simulink model "overcurrent_undervoltag_relay"  (R2025b)
settings: Solver=VariableStepAuto  StartTime=0.0  StopTime=2.00  RelTol=1e-3
libraries: dspstat3 x3, simulink x1
settings Model: Creator=urshi  LastModifiedBy=urshi

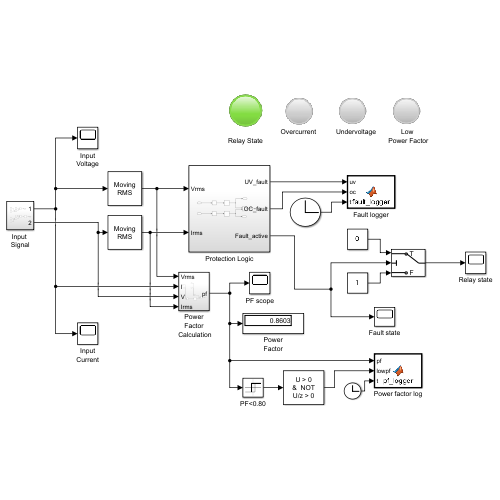
[thumbnail: Simulink's stored preview of the top-level diagram]
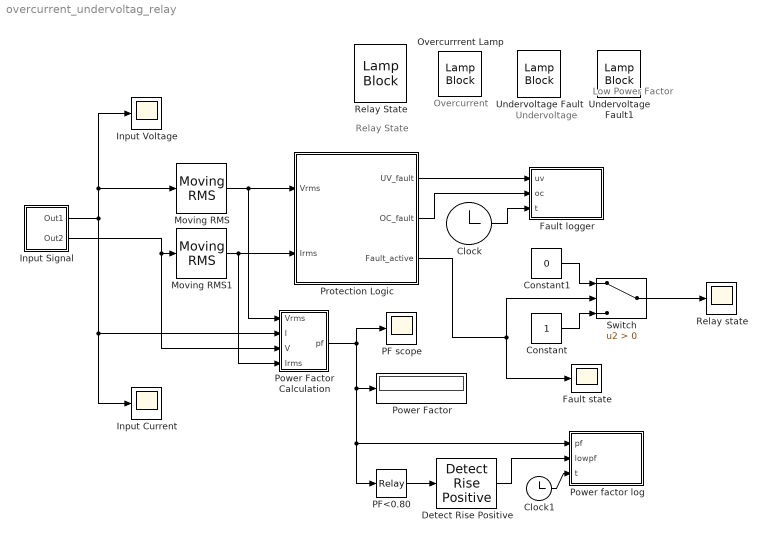
== system overcurrent_undervoltag_relay ==
  note: Low
      | Power Factor
  note: Relay State
  note: Undervoltage
  note: Overcurrent
  Clock : Clock
  Clock1 : Clock
  Constant : Constant
  Constant1 : Constant  Value=0
  Detect Rise Positive : simulink/Logic and Bit Operations/Detect Rise Positive  vinit=0  OutDataTypeStr=boolean
  Fault logger : MATLAB Function  TreatAsAtomicUnit=on
  Fault state : Scope
      settings: ActiveDisplayYMinimum=-6.1678141135617093  ActiveDisplayYMaximum=11.611256622792828  DataLoggingVariableName=ScopeData2
  Input Current : Scope
      settings: ActiveDisplayYMinimum=-1422.9675846946514  ActiveDisplayYMaximum=1324.8355096908929
  Input Voltage : Scope
      settings: ActiveDisplayYMinimum=-1422.9675846946514  ActiveDisplayYMaximum=1324.8355096908929
  Input Signal : Subsystem
  Moving RMS : dspstat3/Moving RMS  Method=Sliding window  ForgettingFactorPort=off  SpecifyWindowLength=on  WindowLength=200  OverlapLength=199  AllowArbitraryInputLength=off  ForgettingFactor=0.9  SimulateUsing=Interpreted execution
  Moving RMS1 : dspstat3/Moving RMS  Method=Sliding window  ForgettingFactorPort=off  SpecifyWindowLength=on  WindowLength=200  OverlapLength=199  AllowArbitraryInputLength=off  ForgettingFactor=0.9  SimulateUsing=Interpreted execution
  Overcurrrent Lamp : LampBlock  LabelPosition=Hide  DefaultColor=[192.0, 192.0, 192.0]
  PF scope : Scope
      settings: ActiveDisplayYMinimum=0.59741062696120162  ActiveDisplayYMaximum=1.1022229106822319  DataLoggingVariableName=ScopeData4
  PF<0.80 : Relay  OnSwitchValue=0.85  OffSwitchValue=0.80  OnOutputValue=0  OffOutputValue=1
  Power Factor : Display
  Power Factor Calculation : Subsystem
  Power factor log : MATLAB Function  TreatAsAtomicUnit=on
  Protection Logic : Subsystem
  Relay State : LampBlock  LabelPosition=Hide  DefaultColor=[192.0, 192.0, 192.0]
  Relay state : Scope
      settings: ActiveDisplayYMinimum=-0.2045815584191954  ActiveDisplayYMaximum=1.4705379923620556  DataLoggingVariableName=ScopeData3
  Switch : Switch  Criteria=u2 > Threshold  SaturateOnIntegerOverflow=off  InputSameDT=off
  Undervoltage Fault : LampBlock  LabelPosition=Hide  DefaultColor=[192.0, 192.0, 192.0]
  Undervoltage Fault1 : LampBlock  LabelPosition=Hide  DefaultColor=[192.0, 192.0, 192.0]
  wires:
  Input Signal/1(Out1) -> Input Voltage/1, Moving RMS/1, Input Current/1, Power Factor Calculation/2(I)
  Moving RMS/1 -> Power Factor Calculation/1(Vrms), Protection Logic/1(Vrms)
  Moving RMS1/1 -> Power Factor Calculation/4(Irms), Protection Logic/2(Irms)
  Protection Logic/1(UV_fault) -> Fault logger/1(uv)
  Protection Logic/2(OC_fault) -> Fault logger/2(oc)
  Clock/1 -> Fault logger/3(t)
  Protection Logic/3(Fault_active) -> Switch/2, Fault state/1
  Constant1/1 -> Switch/1
  Constant/1 -> Switch/3
  Switch/1 -> Relay state/1
  Clock1/1 -> Power factor log/3(t)
  Power Factor Calculation/1(pf) -> Power factor log/1(pf), PF<0.80/1, Power Factor/1, PF scope/1
  Input Signal/2(Out2) -> Power Factor Calculation/3(V), Moving RMS1/1
  Detect Rise Positive/1 -> Power factor log/2(lowpf)
  PF<0.80/1 -> Detect Rise Positive/1

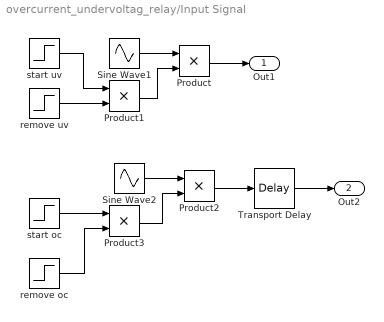
== system overcurrent_undervoltag_relay/Input Signal ==
  Product{,1..3} (4 alike) : Product
  Sine Wave1 : Sin  Amplitude=325.269  Frequency=50*2*pi  SampleTime=0.0002
  Sine Wave2 : Sin  Amplitude=7.071  Frequency=50*2*pi  SampleTime=0.0002
  Transport Delay : TransportDelay  DelayTime=0.00167
  remove oc : Step  Time=0.40  Before=1  After=0.25  SampleTime=0.0002
  remove uv : Step  Time=1.2  Before=1  After=2  SampleTime=0.0002
  start oc : Step  Time=0.15  Before=1  After=4  SampleTime=0.0002
  start uv : Step  Time=0.80  Before=1  After=0.5  SampleTime=0.0002
  Out1 : Outport
  Out2 : Outport  Port=2
  wires:
  remove oc/1 -> Product3/2
  start uv/1 -> Product1/1
  Product3/1 -> Product2/2
  remove uv/1 -> Product1/2
  start oc/1 -> Product3/1
  Product/1 -> Out1/1
  Sine Wave2/1 -> Product2/1
  Sine Wave1/1 -> Product/1
  Product1/1 -> Product/2
  Product2/1 -> Transport Delay/1
  Transport Delay/1 -> Out2/1

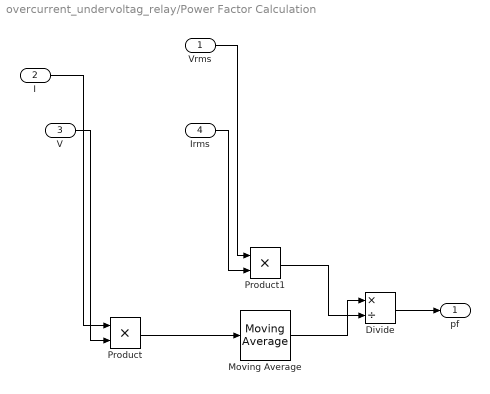
== system overcurrent_undervoltag_relay/Power Factor Calculation ==
  Vrms : Inport
  I : Inport  Port=2
  V : Inport  Port=3
  Irms : Inport  Port=4
  Divide : Product  Inputs=*/
  Moving Average : dspstat3/Moving Average  Method=Sliding window  ForgettingFactorPort=off  SpecifyWindowLength=on  WindowLength=200  OverlapLength=199  AllowArbitraryInputLength=off  ForgettingFactor=0.9  SimulateUsing=Interpreted execution
  Product : Product
  Product1 : Product
  pf : Outport
  wires:
  I/1 -> Product/1
  V/1 -> Product/2
  Divide/1 -> pf/1
  Product/1 -> Moving Average/1
  Moving Average/1 -> Divide/1
  Vrms/1 -> Product1/1
  Irms/1 -> Product1/2
  Product1/1 -> Divide/2

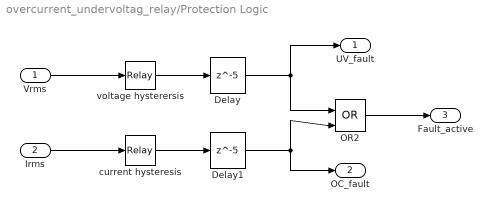
== system overcurrent_undervoltag_relay/Protection Logic ==
  Vrms : Inport
  Irms : Inport  Port=2
  Delay : Delay  DelayLength=5  InputProcessing=Columns as channels (frame based)
  Delay1 : Delay  DelayLength=5  InputProcessing=Columns as channels (frame based)
  OR2 : Logic  Operator=OR  IconShape=distinctive  AllPortsSameDT=off  OutDataTypeStr=boolean
  current hysteresis : Relay  OnSwitchValue=8  OffSwitchValue=7.2
  voltage hysterersis : Relay  OnSwitchValue=190  OffSwitchValue=180  OnOutputValue=0  OffOutputValue=1
  UV_fault : Outport
  OC_fault : Outport  Port=2
  Fault_active : Outport  Port=3
  wires:
  Irms/1 -> current hysteresis/1
  Vrms/1 -> voltage hysterersis/1
  current hysteresis/1 -> Delay1/1
  OR2/1 -> Fault_active/1
  voltage hysterersis/1 -> Delay/1
  Delay/1 -> UV_fault/1, OR2/1
  Delay1/1 -> OR2/2, OC_fault/1

== matlab function overcurrent_undervoltag_relay/Power factor log ==
  data: pf input; lowpf input; t input
function pf_logger(pf, lowpf, t)

persistent prev_lowpf

if isempty(prev_lowpf)
    prev_lowpf = 0;
end

if lowpf && ~prev_lowpf
    fprintf('LOW PF: %.2f at %.2f s\n', pf, t);
end

== matlab function overcurrent_undervoltag_relay/Fault logger ==
  data: uv input; oc input; t input
function fault_logger(uv, oc, t)

persistent fault_active

if isempty(fault_active)
    fault_active = 0;
end

% detect if any fault exists
current_fault = uv || oc;

% FAULT START
if current_fault && fault_active == 0

    if uv && oc
        fprintf('FAULT START: OVERCURRENT + UNDERVOLTAGE at %.2f s\n', t);

    elseif uv
        fprintf('FAULT START: UNDERVOLTAGE at %.2f s\n', t);

    elseif oc
        fprintf('FAULT START: OVERCURRENT at %.2f s\n', t);
    end

    fault_active = 1;
end

% FAULT CLEARED
if ~current_fault && fault_active == 1
    fprintf('FAULT CLEARED at %.2f s\n', t);
    fault_active = 0;
end
